simulink library "gravLoads3D_ul"  (R2020a)
settings: Solver=VariableStepAuto  StartTime=0.0  StopTime=10.0  RelTol=1e-3
undefined symbols (not defined in the file): Env, Veh
libraries: simulink x2, vrlib x1
settings Model: Creator=John Jr  LastModifiedBy=John Jr

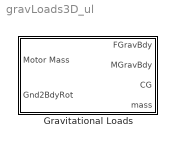
== system gravLoads3D_ul ==
  Gravitational Loads : Subsystem  mask{g=Env.grav.Value, m=Veh.structMass.Value, CG1=Veh.rCMpad_B.Value, CG2=Veh.rCMair_B.Value, t_b=Veh.motor.burnTime.Value}
      mask prompts: g "Gravitational acceleration [m/s^2]"; m "Vehicle mass without motor [kg]"; CG1 "CG on launchpad [m]"; CG2 "CG after motor burn [m]"; t_b "Total motor burn time [s]"
      mask DialogControl DescGroupVar Prompt: Gravitational Force Library
      mask DialogControl DescTextVar Prompt: This block models the gravitational force acting on the vehicle, as well as the stability margin as the motor burns.
      mask DialogControl Control2 Prompt: Stability Properties (measured from nosecone):
      mask Display:
      | patch([0 1 1 0], [0 0 1 1],[.8 1 1])
      | 
      | port_label('input',1,'\fontname{Cambria Math}motorMass','texmode','on')
      | port_label('input',2,'\fontname{Cambria Math}Gnd2BdyRot','texmode','on')
      | 
      | port_label('output',1,'\fontname{Cambria Math}FGravBdy','texmode','on')
      | port_label('output',2,'\fontname{Cambria Math}MGravBdy','texmode','on')
      | port_label('output',3,'\fontname{Cambria Math}rCM_B','texmode','on')
      | port_label('output',4,'\fontname{Cambria Math}mass','texmode','on')

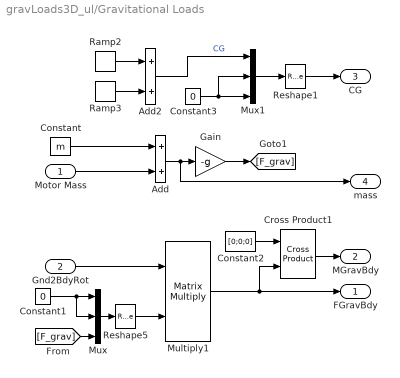
== system gravLoads3D_ul/Gravitational Loads ==
  Motor Mass : Inport
  Gnd2BdyRot : Inport  Port=2
  Add : Sum
  Add2 : Sum
  Constant : Constant  Value=m
  Constant1 : Constant  Value=0
  Constant2 : Constant  Value=[0;0;0]
  Constant3 : Constant  Value=0
  Cross Product1 : vrlib/Utilities/Cross Product
  Gain : Gain  Gain=-g
  Multiply1 : Product  Multiplication=Matrix(*)
  Mux : Mux  Inputs=3
  Mux1 : Mux  Inputs=3
  Ramp2 : simulink/Sources/Ramp  slope=-(CG1(1)-CG2(1))/t_b  start=0  InitialOutput=CG1(1)
  Ramp3 : simulink/Sources/Ramp  slope=(CG1(1)-CG2(1))/t_b  start=t_b  InitialOutput=0
  Reshape1 : Reshape  OutputDimensionality=Column vector (2-D)
  Reshape5 : Reshape  OutputDimensionality=Column vector (2-D)
  FGravBdy : Outport  VectorParamsAs1DForOutWhenUnconnected=off
  MGravBdy : Outport  Port=2  VectorParamsAs1DForOutWhenUnconnected=off
  CG : Outport  Port=3  VectorParamsAs1DForOutWhenUnconnected=off
  mass : Outport  Port=4  VectorParamsAs1DForOutWhenUnconnected=off
  wires:
  Gain/1 -> [F_grav]
  Ramp2/1 -> Add2/1
  Ramp3/1 -> Add2/2
  Constant/1 -> Add/1
  Add/1 -> mass/1, Gain/1
  Motor Mass/1 -> Add/2
  Constant1/1 -> Mux/1, Mux/2
  [F_grav] -> Mux/3
  Mux/1 -> Reshape5/1
  Reshape5/1 -> Multiply1/2
  Gnd2BdyRot/1 -> Multiply1/1
  Multiply1/1 -> Cross Product1/2, FGravBdy/1
  Cross Product1/1 -> MGravBdy/1
  Constant2/1 -> Cross Product1/1
  Reshape1/1 -> CG/1
  Mux1/1 -> Reshape1/1
  Constant3/1 -> Mux1/2, Mux1/3
  Add2/1 -> Mux1/1  "CG"
